simulink model "DisplayControl"  (R2015a)
settings: configuration reference "config_cosim" (kept outside this file)
settings Model: CovModelRefEnable=off  Creator=zhang  LastModifiedBy=yrzhang
settings ConfigSetRef: SourceLocation=Base Workspace

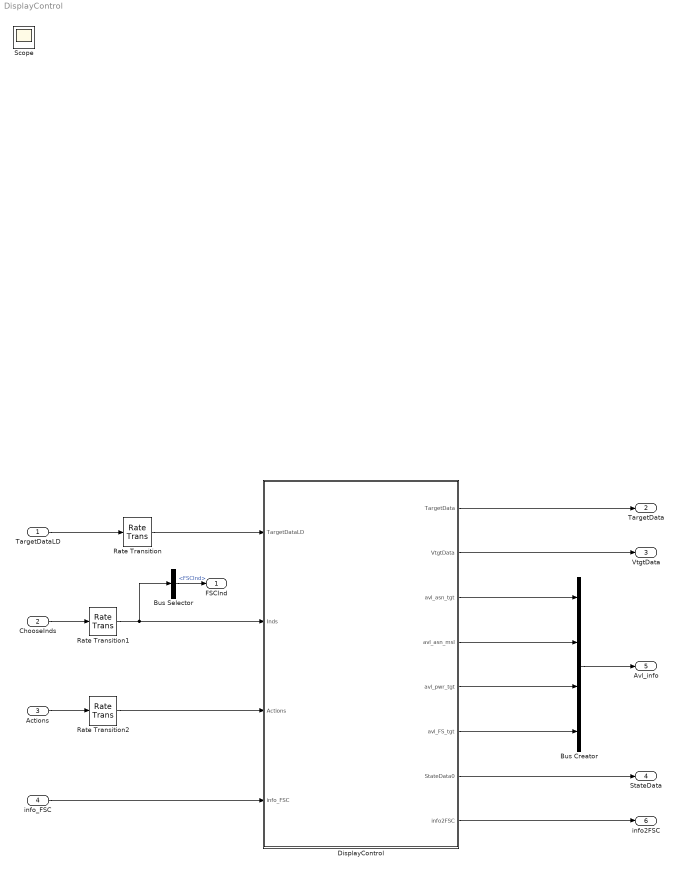
== system DisplayControl ==
  TargetDataLD : Inport  OutDataTypeStr=Bus: TgtDataLDBusObject
  ChooseInds : Inport  Port=2  OutDataTypeStr=Bus:ChooseBusObject
  Actions : Inport  Port=3  OutDataTypeStr=Bus: ActionBusObject
  info_FSC : Inport  Port=4  OutDataTypeStr=Bus:BusObject_info_FSC2CC
  Bus Creator : BusCreator  OutDataTypeStr=Bus:AvlBusObject
  Bus Selector : BusSelector  OutputSignals=FSCInd
  DisplayControl : Stateflow chart  TreatAsAtomicUnit=on
  Rate Transition : RateTransition
  Rate Transition1 : RateTransition
  Rate Transition2 : RateTransition
  FSCInd : Outport
  TargetData : Outport  Port=2
  VtgtData : Outport  Port=3
  StateData : Outport  Port=4  OutDataTypeStr=Bus:StateBusObject
  Avl_info : Outport  Port=5  OutDataTypeStr=Bus:AvlBusObject
  info2FSC : Outport  Port=6  OutDataTypeStr=Bus: BusObject_info_CC2FSC
  Scope : Scope
  wires:
  TargetDataLD/1 -> Rate Transition/1
  ChooseInds/1 -> Rate Transition1/1
  Bus Selector/1 -> FSCInd/1  "<FSCInd>"
  Actions/1 -> Rate Transition2/1
  DisplayControl/3(avl_asn_tgt) -> Bus Creator/1
  DisplayControl/5(avl_pwr_tgt) -> Bus Creator/3
  DisplayControl/6(avl_FS_tgt) -> Bus Creator/4
  Rate Transition/1 -> DisplayControl/1(TargetDataLD)
  DisplayControl/8(info2FSC) -> info2FSC/1
  Bus Creator/1 -> Avl_info/1
  DisplayControl/1(TargetData) -> TargetData/1
  DisplayControl/7(StateData0) -> StateData/1
  Rate Transition2/1 -> DisplayControl/3(Actions)
  info_FSC/1 -> DisplayControl/4(info_FSC)
  DisplayControl/4(avl_asn_msl) -> Bus Creator/2
  Rate Transition1/1 -> DisplayControl/2(Inds), Bus Selector/1
  DisplayControl/2(VtgtData) -> VtgtData/1

== stateflow chart DisplayControl/DisplayControl ==
  settings: executeAtInitialization=1
  state Init
    entry:
    TargetData(:,1) = TargetDataLD.L;
    TargetData(:,3) = TargetDataLD.H;
    VtgtData = TargetDataLD.V;
    TargetData(:,7) = TargetDataLD.Index;
    StateData = zeros(8,3);
    StateInf = 0;
    avl_asn_msl = ones(8,1);
    avl_FS_tgt = zeros(8,1);
    avl_pwr_tgt = zeros(8,1);
  state On
    state TargetPower [parallel]
      % 根据选择的目标更新加电和断电信息
      settings: executionOrder=4
      TargetPower -> (junction 337)
      (junction 337) -> (junction 441) [order 1] : [Actions.TgtAsn]
      (junction 337) -> (junction 339) [order 2]
      (junction 441) -> (junction 443) : {avl_pwr_tgt(Inds.TgtAsnInd) = 1;}
      (junction 443) -> (junction 339)
      (junction 339) -> (junction 687)
      (junction 687) -> (junction 685) [order 1] : [Actions.TgtAsnCcl]
      (junction 687) -> (junction 684) [order 2]
      (junction 685) -> (junction 691) : {avl_pwr_tgt(Inds.TgtAsnInd) = 0;}
      (junction 691) -> (junction 684)
    state DataProcess [parallel]
      en:
      %info2FSC.Para_FS(1:8) = 0;
      Para_FS0.pos_tgt = [0;0;0];
      Para_FS0.vel_tgt = [0;0;0];
      info2FSC.Para_FS(1:8) = Para_FS0;
      info2FSC.ins_pwr_on =  false(8,1);
      info2FSC.ins_pwr_of = [false;false;false;false;false;false;false;false];
      info2FSC.ins_FS = [false;false;false;false;false;false;false;false];
      settings: executionOrder=6
      state PwrOff [parallel]
        settings: executionOrder=3
        (default) -> (junction 889)
        PwrOff -> (junction 889)
        (junction 889) -> (junction 880) [order 1] : [Actions.PwrOff]
        (junction 889) -> (junction 877) [order 2]
        (junction 880) -> (junction 885) : {info2FSC.ins_pwr_on = [false;false;false;false;false;false;false;false];
            | info2FSC.ins_pwr_of = [false;false;false;false;false;false;false;false];
            | info2FSC.ins_FS = [false;false;false;false;false;false;false;false];}
        (junction 885) -> (junction 877)
        (junction 877) -> (junction 1217) : {i = 1;}
        (junction 888) -> (junction 897) [order 1] : [Inds.TgtPwrInd(i,1)]
        (junction 1217) -> (junction 888) [order 1] : [i  < 8]
        (junction 888) -> (junction 882) [order 2]
        (junction 897) -> (junction 1197) : {ddInd1 = TargetData(i,5);
            | info2FSC.ins_pwr_of(ddInd1) = true;}
        (junction 1197) -> (junction 882)
        (junction 891) -> (junction 1217) : {i = i + 1;}
        (junction 1217) -> (junction 1219) [order 2]
        (junction 882) -> (junction 894)
        (junction 894) -> (junction 893) [order 1] : [Inds.TgtPwrInd(i,2)]
        (junction 894) -> (junction 891) [order 2]
        (junction 893) -> (junction 1199) : {ddInd1 = TargetData(i,6);
            | info2FSC.ins_pwr_of(ddInd1) = true;}
        (junction 1199) -> (junction 891)
      state PwrOn [parallel]
        settings: executionOrder=1
        (default) -> (junction 863)
        PwrOn -> (junction 863)
        (junction 863) -> (junction 852) [order 1] : [Actions.PwrOn]
        (junction 863) -> (junction 853) [order 2]
        (junction 852) -> (junction 851) : {info2FSC.ins_pwr_on = [false;false;false;false;false;false;false;false];
            | info2FSC.ins_pwr_of = [false;false;false;false;false;false;false;false];
            | info2FSC.ins_FS = [false;false;false;false;false;false;false;false];}
        (junction 851) -> (junction 853)
        (junction 862) -> (junction 864) [order 1] : [Inds.TgtPwrInd(i,1)]
        (junction 1214) -> (junction 862) [order 1] : [i  < 8]
        (junction 853) -> (junction 1214) : {i = 1;}
        (junction 862) -> (junction 857) [order 2]
        (junction 864) -> (junction 1193) : {ddInd1 = TargetData(i,5);
            | info2FSC.ins_pwr_on(ddInd1) = true;}
        (junction 1193) -> (junction 857)
        (junction 857) -> (junction 870)
        (junction 869) -> (junction 1214) : {i = i + 1;}
        (junction 1214) -> (junction 1212) [order 2]
        (junction 870) -> (junction 871) [order 1] : [Inds.TgtPwrInd(i,2)]
        (junction 870) -> (junction 869) [order 2]
        (junction 871) -> (junction 1195) : {ddInd1 = TargetData(i,6);
            | info2FSC.ins_pwr_on(ddInd1) = true;}
        (junction 1195) -> (junction 869)
      state FS [parallel]
        settings: executionOrder=2
        (default) -> (junction 914)
        On.DataProcess.FS -> (junction 914)
        (junction 914) -> (junction 905) [order 1] : [Actions.FS]
        (junction 914) -> (junction 902) [order 2]
        (junction 905) -> (junction 910) : {info2FSC.ins_pwr_on = [false;false;false;false;false;false;false;false];
            | info2FSC.ins_pwr_of = [false;false;false;false;false;false;false;false];
            | info2FSC.ins_FS = [false;false;false;false;false;false;false;false];}
        (junction 910) -> (junction 902)
        (junction 902) -> (junction 1221) : {i = 1;}
        (junction 913) -> (junction 922) [order 1] : [Inds.TgtFsInd(i,1)]
        (junction 1221) -> (junction 913) [order 1] : [i  < 8]
        (junction 913) -> (junction 907) [order 2]
        (junction 922) -> (junction 1201) : {ddInd1 = TargetData(i,5);
            | info2FSC.ins_FS(ddInd1) = true;}
        (junction 1201) -> (junction 907)
        (junction 907) -> (junction 919)
        (junction 916) -> (junction 1221) : {i = i + 1;}
        (junction 1221) -> (junction 1222) [order 2]
        (junction 919) -> (junction 918) [order 1] : [Inds.TgtFsInd(i,2)]
        (junction 918) -> (junction 1203) : {ddInd1 = TargetData(i,6);
            | info2FSC.ins_FS(ddInd1) = true;}
        (junction 919) -> (junction 916) [order 2]
        (junction 1203) -> (junction 916)
      state DataUpdateWithFSCInfo [parallel]
        settings: executionOrder=4
        (default) -> (junction 981) : {avl_asn_msl =double(avl_asn_msl&info_FSC.avl_msl);}
        DataUpdateWithFSCInfo -> (junction 981)
        (junction 981) -> (junction 980) : {m = 0;
            | n = 0;
            | j = 1;}
        (junction 979) -> (junction 968) [order 1] : % 导弹出现故障
            | [~info_FSC.avl_msl(j)]
        (junction 980) -> (junction 979) [order 1] : [j  < 8]
        (junction 979) -> (junction 972) [order 2]
        (junction 968) -> (junction 994) : {StateData(j,1:3) =2;}
        (junction 972) -> (junction 984) [order 1] : %虽然有加电命令，但是加电状态为未加电
            | [info2FSC.ins_pwr_on(j)==1 && info_FSC.stt_pwr_msl(j) ==0]
        (junction 977) -> (junction 980) : {j = j + 1;}
        (junction 980) -> (junction 1177) [order 2]
        (junction 972) -> (junction 973) [order 2]
        (junction 984) -> (junction 988) : {StateData(j,2) = 0;
            | m = m+1;}
        (junction 973) -> (junction 966) [order 1] : %虽然有发射命令，但是离架计时为0，说明没有发生
            | [info2FSC.ins_FS(j)==1 && info_FSC.count_sprt_msl(j)<=0]
        (junction 973) -> (junction 977) [order 2]
        (junction 966) -> (junction 991) : {StateData(j,3) = 0;
            | n = n+1;}
        (junction 991) -> (junction 977)
        (junction 988) -> (junction 991)
        (junction 994) -> (junction 988)
        (junction 1177) -> (junction 1173) [order 1] : [Actions.PwrOn||Actions.PwrOff||Actions.FS]
        (junction 1177) -> (junction 1174) [order 2]
        (junction 1173) -> (junction 1178) : {StateInf = 0;}
        (junction 1178) -> (junction 1174)
        (junction 1174) -> (junction 999)
        (junction 999) -> (junction 1001) [order 1] : [sum(info2FSC.ins_pwr_on)>0&&m == sum(info2FSC.ins_pwr_on)] % 说明本次没有加电成功的DD
        (junction 999) -> (junction 1005) [order 2]
        (junction 1001) -> (junction 1003) : {StateInf = 712;}
        (junction 1003) -> (junction 1005)
        (junction 1005) -> (junction 1009)
        (junction 1009) -> (junction 1011) [order 1] : [sum(info2FSC.ins_FS)>0&&n == sum(info2FSC.ins_FS)] % 说明本次没有发射成功的DD
        (junction 1009) -> (junction 1008) [order 2]
        (junction 1011) -> (junction 1012) : {StateInf = 110;}
        (junction 1012) -> (junction 1008)
        (junction 1008) -> (junction 1021) : {StateData0.StateData = StateData;
            | StateData0.StateInf = StateInf;
            | j = 1;}
        (junction 1024) -> (junction 1040) [order 1] : [avl_FS_tgt(j) == 1]
        (junction 1040) -> (junction 1086) [order 1] : % 选了j个目标的第1颗dd
            | [Inds.TgtPwrInd(j,1)]
        (junction 1021) -> (junction 1024) [order 1] : [j<8]
        (junction 1024) -> (junction 1208) [order 2]
        (junction 1040) -> (junction 1098) [order 2] : {DD1 = 0;
            | DD10 = 0; }
        (junction 1086) -> (junction 1088) : %j个目标的第一颗dd编号
            | {DD1 = TargetData(j,5);}
        (junction 1088) -> (junction 1098)
        (junction 1098) -> (junction 1106)
        (junction 1106) -> (junction 1104) [order 1] : [DD1>0]
        (junction 1104) -> (junction 1105) [order 1] : %这颗dd的状态为0
            | [info_FSC.stt_pwr_msl(DD1)==0]
        (junction 1106) -> (junction 1110) [order 2]
        (junction 1104) -> (junction 1141) [order 2] : {DD10 = 1;}
        (junction 1105) -> (junction 1112) : %选中了dd1且dd1状态为0
            | {DD10 = 0;}
        (junction 1141) -> (junction 1110)
        (junction 1112) -> (junction 1141)
        (junction 1110) -> (junction 1092)
        (junction 1208) -> (junction 1021) : {j = j+1;}
        (junction 1021) -> (junction 1034) [order 2]
        (junction 1092) -> (junction 1096) [order 1] : [Inds.TgtPwrInd(j,2)]
        (junction 1092) -> (junction 1101) [order 2] : {DD2 = 0;
            | DD20= 0;}
        (junction 1096) -> (junction 1094) : {DD2 = TargetData(j,6);}
        (junction 1094) -> (junction 1101)
        (junction 1101) -> (junction 1125)
        (junction 1125) -> (junction 1126) [order 1] : [DD2>0]
        (junction 1126) -> (junction 1127) [order 1] : [info_FSC.stt_pwr_msl(DD2)==0]
        (junction 1125) -> (junction 1118) [order 2]
        (junction 1126) -> (junction 1143) [order 2] : {DD20 = 1;}
        (junction 1127) -> (junction 1122) : {DD20 = 0;}
        (junction 1143) -> (junction 1118)
        (junction 1122) -> (junction 1143)
        (junction 1118) -> (junction 1036)
        (junction 1036) -> (junction 1048) [order 1] : % 两颗dd均被选，但是两颗dd的状态均为0
            | % 或者一颗dd选中了，其状态为0，而另一颗dd未选
            | [DD10==0&&DD20==0]
        (junction 1036) -> (junction 1138) [order 2]
        (junction 1048) -> (junction 1137) : {avl_FS_tgt(j) = 0;}
        (junction 1138) -> (junction 1208)
        (junction 1137) -> (junction 1138)
    state TargetDataProcess [parallel]
      settings: executionOrder=1
      state Time
      (default) -> Time : {TargetData(:,1) = TargetDataLD.L;
          | TargetData(:,3) = TargetDataLD.H;
          | VtgtData = TargetDataLD.V;
          | TargetData(:,7) = TargetDataLD.Index;}
      Time -> TargetDataProcess : [after(1,sec)]
    state DataUpdate [parallel]
      % 根据状态更新状态信息以及表格中要显示的数据
      en:StateData = zeros(8,3);
      settings: executionOrder=2
      state FS [parallel]
        settings: executionOrder=3
        (junction 611) -> (junction 604) [order 1] : [i  < 8]
        (junction 604) -> (junction 607)
        On.DataUpdate.FS -> (junction 605)
        (junction 605) -> (junction 606) [order 1] : [Actions.FS]
        (junction 605) -> (junction 812) [order 2]
        (junction 606) -> (junction 611) : {i = 1;}
        (junction 607) -> (junction 608) [order 1] : [Inds.TgtFsInd(i,1)>0]
        (junction 607) -> (junction 609) [order 2]
        (junction 608) -> (junction 610) : {ddInd = TargetData(i,5);
            | StateData(ddInd,3) = 1;}
        (junction 610) -> (junction 609)
        (junction 609) -> (junction 612)
        (junction 617) -> (junction 611) : {i = i + 1;}
        (junction 611) -> (junction 616) [order 2]
        (junction 612) -> (junction 613) [order 1] : [Inds.TgtFsInd(i,2)>0]
        (junction 612) -> (junction 614) [order 2]
        (junction 613) -> (junction 615) : {ddInd = TargetData(i,6);
            | StateData(ddInd,3) = 1;}
        (junction 615) -> (junction 614)
        (junction 812) -> (junction 616)
        (junction 614) -> (junction 617)
      state Assign [parallel]
        settings: executionOrder=1
        Assign -> (junction 412)
        (junction 412) -> (junction 416) [order 1] : [Inds.TgtAsnInd>0&&Actions.TgtAsn]
        (junction 412) -> (junction 415) [order 2]
        (junction 416) -> (junction 410) : {TargetData(Inds.TgtAsnInd,5) = ((Inds.FSCInd-1)*2+1)*Inds.MslInd(1);
            |  TargetData(Inds.TgtAsnInd,6) = ((Inds.FSCInd-1)*2+2)*Inds.MslInd(2);}
        (junction 410) -> (junction 447) [order 1] : [Inds.MslInd(1)]
        (junction 410) -> (junction 815) [order 2]
        (junction 447) -> (junction 814) : {StateData((Inds.FSCInd-1)*2+1,1) = 1;}
        (junction 814) -> (junction 815)
        (junction 815) -> (junction 449)
        (junction 449) -> (junction 452) [order 1] : [Inds.MslInd(2)]
        (junction 449) -> (junction 454) [order 2]
        (junction 452) -> (junction 818) : {StateData((Inds.FSCInd-1)*2+2,1) = 1;}
        (junction 454) -> (junction 415)
        (junction 818) -> (junction 454)
        (junction 415) -> (junction 662)
        (junction 662) -> (junction 664) [order 1] : [Inds.TgtAsnInd>0&&Actions.TgtAsnCcl]
        (junction 664) -> (junction 679) [order 1] : [Inds.FSCInd]
        (junction 662) -> (junction 665) [order 2]
        (junction 664) -> (junction 676) [order 2]
        (junction 679) -> (junction 820) : {TargetData(Inds.TgtAsnInd,5) = 0;
            |  TargetData(Inds.TgtAsnInd,6) = 0;
            | StateData((Inds.FSCInd-1)*2+1,1) = 0;
            | StateData((Inds.FSCInd-1)*2+2,1) = 0;}
        (junction 676) -> (junction 665)
        (junction 820) -> (junction 676)
      state Pwr [parallel]
        settings: executionOrder=2
        (junction 532) -> (junction 530) [order 1] : [i  < 8]
        (junction 530) -> (junction 544)
        (junction 544) -> (junction 543) [order 1] : [Inds.TgtPwrInd(i,1)>0]
        (junction 544) -> (junction 545) [order 2]
        (junction 543) -> (junction 542) : {ddInd = TargetData(i,5);
            | StateData(ddInd,2) = 1;}
        (junction 542) -> (junction 545)
        (junction 545) -> (junction 559)
        Pwr -> (junction 484)
        (junction 484) -> (junction 531) [order 1] : [Actions.PwrOn]
        (junction 559) -> (junction 553) [order 1] : [Inds.TgtPwrInd(i,2)>0]
        (junction 484) -> (junction 809) [order 2]
        (junction 531) -> (junction 532) : {i = 1;}
        (junction 559) -> (junction 554) [order 2]
        (junction 553) -> (junction 552) : {ddInd = TargetData(i,6);
            | StateData(ddInd,2) = 1;}
        (junction 552) -> (junction 554)
        (junction 554) -> (junction 533)
        (junction 735) -> (junction 718) [order 1] : [i  < 8]
        (junction 718) -> (junction 728)
        (junction 533) -> (junction 532) : {i = i + 1;}
        (junction 532) -> (junction 534) [order 2]
        (junction 728) -> (junction 727) [order 1] : [Inds.TgtPwrInd(i,1)>0]
        (junction 728) -> (junction 719) [order 2]
        (junction 727) -> (junction 725) : {ddInd = TargetData(i,5);
            | StateData(ddInd,2) = 0;}
        (junction 534) -> (junction 716) [order 1] : [Actions.PwrOff]
        (junction 809) -> (junction 534)
        (junction 725) -> (junction 719)
        (junction 534) -> (junction 808) [order 2]
        (junction 716) -> (junction 735) : {i = 1;}
        (junction 719) -> (junction 723)
        (junction 723) -> (junction 733) [order 1] : [Inds.TgtPwrInd(i,2)>0]
        (junction 723) -> (junction 724) [order 2]
        (junction 733) -> (junction 721) : {ddInd = TargetData(i,6);
            | StateData(ddInd,2) = 0;}
        (junction 721) -> (junction 724)
        (junction 724) -> (junction 732)
        (junction 732) -> (junction 735) : {i = i + 1;}
        (junction 735) -> (junction 744) [order 2]
        (junction 808) -> (junction 744)
    state TargetAssign [parallel]
      % 根据选择的目标、FSC和DD更新可分配的目标、FSC和DD数据
      en:avl_asn_tgt = ones(8,1);
      settings: executionOrder=3
      (junction 328) -> (junction 330) [order 1] : [Actions.TgtAsn]
      TargetAssign -> (junction 328)
      (junction 330) -> (junction 421) : {avl_asn_tgt(Inds.TgtAsnInd) = 0;}
      (junction 328) -> (junction 329) [order 2]
      (junction 421) -> (junction 423) [order 1] : [Inds.MslInd(1)>0]
      (junction 421) -> (junction 824) [order 2]
      (junction 423) -> (junction 826) : {avl_asn_msl((Inds.FSCInd-1)*2+1) = 0;}
      (junction 826) -> (junction 824)
      (junction 824) -> (junction 430)
      (junction 430) -> (junction 436) [order 1] : [Inds.MslInd(2)>0]
      (junction 430) -> (junction 434) [order 2]
      (junction 436) -> (junction 822) : {avl_asn_msl((Inds.FSCInd-1)*2+2) = 0;}
      (junction 434) -> (junction 329)
      (junction 822) -> (junction 434)
      (junction 329) -> (junction 637)
      (junction 637) -> (junction 655) [order 1] : [Actions.TgtAsnCcl]
      (junction 655) -> (junction 641) : {avl_asn_tgt(Inds.TgtAsnInd) = 1;}
      (junction 637) -> (junction 639) [order 2]
      (junction 641) -> (junction 647) [order 1] : [Inds.MslInd(1)>0]
      (junction 641) -> (junction 831) [order 2]
      (junction 647) -> (junction 830) : {avl_asn_msl((Inds.FSCInd-1)*2+1) = 1;}
      (junction 830) -> (junction 831)
      (junction 831) -> (junction 646)
      (junction 646) -> (junction 648) [order 1] : [Inds.MslInd(2)>0]
      (junction 648) -> (junction 828) : {avl_asn_msl((Inds.FSCInd-1)*2+2) = 1;}
      (junction 646) -> (junction 643) [order 2]
      (junction 643) -> (junction 639)
      (junction 828) -> (junction 643)
    state FS [parallel]
      % 根据选择的目标更新DD发射信息
      settings: executionOrder=5
      On.FS -> (junction 587)
      (junction 587) -> (junction 585) [order 1] : [Actions.PwrOn]
      (junction 587) -> (junction 693) [order 2]
      (junction 585) -> (junction 577) : {i = 1;}
      (junction 577) -> (junction 693) [order 2]
      (junction 577) -> (junction 590) [order 1] : [i  < 8]
      (junction 590) -> (junction 597) [order 1] : [Inds.TgtPwrInd(i,1)||Inds.TgtPwrInd(i,2)]
      (junction 571) -> (junction 577) : {i = i + 1;}
      (junction 693) -> (junction 707)
      (junction 590) -> (junction 571) [order 2]
      (junction 597) -> (junction 1185) : {avl_FS_tgt(i) = 1;}
      (junction 1185) -> (junction 571)
      (junction 707) -> (junction 700) [order 1] : [Actions.PwrOff]
      (junction 707) -> (junction 708) [order 2]
      (junction 700) -> (junction 704) : {i = 1;}
      (junction 704) -> (junction 708) [order 2]
      (junction 704) -> (junction 771) [order 1] : [i  < 8]
      (junction 771) -> (junction 770) [order 1] : [Inds.TgtPwrInd(i,1)]
      (junction 796) -> (junction 704) : {i = i + 1;}
      (junction 771) -> (junction 747) [order 2]
      (junction 770) -> (junction 777) : %该目标的配置的另一个DD
          | {ddInd = TargetData(i,6);}
      (junction 777) -> (junction 798) [order 1] : [ddInd==0||(ddInd~=0&&StateData(ddInd,2) == 0)]
      (junction 777) -> (junction 778) [order 2]
      (junction 798) -> (junction 1187) : {avl_FS_tgt(i) = 0;}
      (junction 778) -> (junction 747)
      (junction 1187) -> (junction 778)
      (junction 747) -> (junction 754)
      (junction 754) -> (junction 769) [order 1] : [Inds.TgtPwrInd(i,2)]
      (junction 754) -> (junction 796) [order 2]
      (junction 769) -> (junction 788) : {ddInd = TargetData(i,5);}
      (junction 788) -> (junction 804) [order 1] : [ddInd==0||(ddInd~=0&&StateData(ddInd,1) == 0)]
      (junction 788) -> (junction 1189) [order 2]
      (junction 804) -> (junction 806) : {avl_FS_tgt(i) = 0;}
      (junction 1189) -> (junction 796)
      (junction 806) -> (junction 1189)
  (default) -> Init
  Init -> On : after(1,sec)
  data: TargetDataLD input Bus: TgtDataLDBusObject size=1; Inds input Bus: ChooseBusObject size=1; TargetData output double size=[8 7]; VtgtData output size=[8 3]; avl_asn_tgt output double size=8; avl_asn_msl output double size=8; avl_pwr_tgt output double size=8; avl_FS_tgt output double size=8; StateData0 output Bus: StateBusObject; i local; ddInd local; info2FSC output Bus: BusObject_info_CC2FSC size=1; ddInd1 local; Actions input Bus: ActionBusObject size=1; info_FSC input Bus: BusObject_info_FSC2CC size=1; StateData local double size=[8 3]; StateInf local double size=1; m local; n local; j local; DD1 local; DD2 local; Para_FS0 local Bus: BusObject_msg_FSC2msl; DD10 local; DD20 local
